simulink model "ApproachControl"  (R2018b)
settings: configuration reference "RPi_ControlRate" (kept outside this file)
values from neighbouring files (symbols this model uses):
  rangeSensorAngBody = [0; 90*dtr; 180*dtr; 270*dtr]    [loadSensorData.m]
libraries: simulink x1
settings Model: Creator=barthal  LastModifiedBy=barthal
settings ConfigSetRef: SourceLocation=Base Workspace

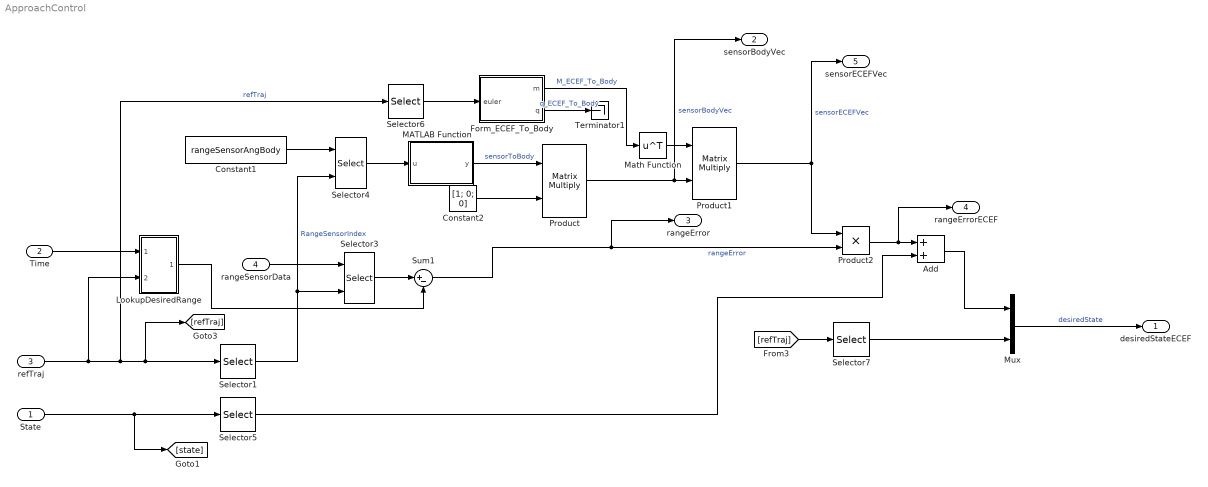
== system ApproachControl ==
  State : Inport  OutDataTypeStr=double
  Time : Inport  Port=2  PortDimensions=1
  refTraj : Inport  Port=3  OutDataTypeStr=double  PortDimensions=[6 15]
  rangeSensorData : Inport  Port=4  OutDataTypeStr=double
  Add : Sum
  Constant1 : Constant  Value=rangeSensorAngBody
  Constant2 : Constant  Value=[1; 0; 0]
  Form_ECEF_To_Body : MATLAB Function  TreatAsAtomicUnit=on
  LookupDesiredRange : Subsystem
  MATLAB Function : MATLAB Function  TreatAsAtomicUnit=on
  Math Function : Math  Operator=transpose  SaturateOnIntegerOverflow=on
  Mux : Mux  Inputs=2
  Product : Product  Multiplication=Matrix(*)
  Product1 : Product  Multiplication=Matrix(*)
  Product2 : Product
  Selector1 : Selector  NumberOfDimensions=2  InputPortWidth=3  IndexOptions=Index vector (dialog),Index vector (dialog)  Indices=6,14  OutputSizes=1,1
  Selector3 : Selector  InputPortWidth=4  IndexOptions=Index vector (port)  Indices=5  OutputSizes=1
  Selector4 : Selector  InputPortWidth=4  IndexOptions=Index vector (port)  Indices=5  OutputSizes=1
  Selector5 : Selector  InputPortWidth=12  IndexOptions=Index vector (dialog)  Indices=[1:3]  OutputSizes=1
  Selector6 : Selector  NumberOfDimensions=2  InputPortWidth=3  IndexOptions=Index vector (dialog),Index vector (dialog)  Indices=6,[5:7]  OutputSizes=1,1
  Selector7 : Selector  NumberOfDimensions=2  InputPortWidth=3  IndexOptions=Index vector (dialog),Index vector (dialog)  Indices=6,[5:13]  OutputSizes=1,1
  Sum1 : Sum  Inputs=|+-
  Terminator1 : Terminator
  desiredStateECEF : Outport
  sensorBodyVec : Outport  Port=2
  rangeError : Outport  Port=3
  rangeErrorECEF : Outport  Port=4
  sensorECEFVec : Outport  Port=5
  wires:
  refTraj/1 -> LookupDesiredRange/2(refTraj), [refTraj], Selector1/1, Selector6/1  "refTraj"
  Time/1 -> LookupDesiredRange/1(Time)
  State/1 -> [state], Selector5/1
  Selector1/1 -> Selector4/2, Selector3/2  "RangeSensorIndex"
  rangeSensorData/1 -> Selector3/1
  Selector3/1 -> Sum1/1
  Sum1/1 -> rangeError/1, Product2/2  "rangeError"
  Constant1/1 -> Selector4/1
  Selector4/1 -> MATLAB Function/1(u)
  MATLAB Function/1(y) -> Product/1  "sensorToBody"
  Constant2/1 -> Product/2
  Product/1 -> sensorBodyVec/1, Product1/2  "sensorBodyVec"
  Product1/1 -> Product2/1, sensorECEFVec/1  "sensorECEFVec"
  Selector5/1 -> Add/2
  Product2/1 -> rangeErrorECEF/1, Add/1
  Add/1 -> Mux/1
  LookupDesiredRange/1(DesiredRange) -> Sum1/2
  Selector6/1 -> Form_ECEF_To_Body/1(euler)
  Selector7/1 -> Mux/2
  [refTraj] -> Selector7/1
  Mux/1 -> desiredStateECEF/1  "desiredState"
  Form_ECEF_To_Body/2(q) -> Terminator1/1  "q_ECEF_To_Body"
  Form_ECEF_To_Body/1(m) -> Math Function/1  "M_ECEF_To_Body"
  Math Function/1 -> Product1/1

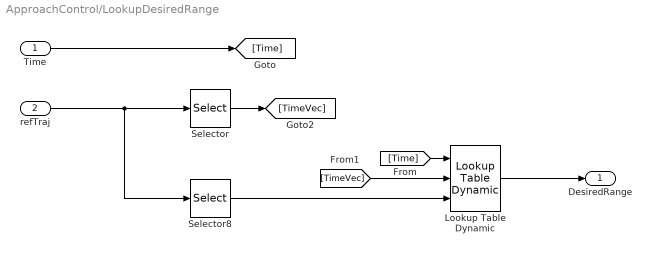
== system ApproachControl/LookupDesiredRange ==
  Time : Inport
  refTraj : Inport  Port=2
  Lookup Table Dynamic : simulink/Lookup Tables/Lookup Table Dynamic  LookUpMeth=Interpolation-Use End Values  OutDataType=fixdt('double')  OutScaling=[]  OutputDataTypeScalingMode=Specify via dialog  OutDataTypeStr=double  DoSatur=off
      settings: SourceProductName=Simulink
  Selector : Selector  NumberOfDimensions=2  InputPortWidth=3  IndexOptions=Select all,Index vector (dialog)  Indices=1,1  OutputSizes=1,1
  Selector8 : Selector  NumberOfDimensions=2  InputPortWidth=3  IndexOptions=Select all,Index vector (dialog)  Indices=1,15  OutputSizes=1,1
  DesiredRange : Outport
  wires:
  Selector8/1 -> Lookup Table Dynamic/3
  [Time] -> Lookup Table Dynamic/1
  [TimeVec] -> Lookup Table Dynamic/2
  Time/1 -> [Time]
  Selector/1 -> [TimeVec]
  refTraj/1 -> Selector8/1, Selector/1
  Lookup Table Dynamic/1 -> DesiredRange/1

== matlab function ApproachControl/MATLAB Function ==
  data: u input; y output
function y = fcn(u)

y = [cos(u) sin(u) 0; -sin(u) cos(u) 0; 0 0 1];

== matlab function ApproachControl/Form_ECEF_To_Body ==
  data: euler input; m output; q output
function [m,q] = fcn(euler)

m = EulerToDCM_321(euler);
q = EulerToquat_321(euler);
